simulink model "mavsim_chap5"  (R2016a)
settings: Solver=ode45  StartTime=0.0  StopTime=10000  RelTol=1e-3
InitFcn:
  | param
values from neighbouring files (symbols this model uses):
  P = GenCoefs(P)    [param.m]    (also in param_chap5.m)
undefined symbols (not defined in the file or in its folder): airdata, drawAircraft, forces_moments, plotmavstatevariables, u_trim
settings Model: Creator=beard  LastModifiedBy=Brian Jackson
settings DataIOCC: LimitDataPoints=on  SaveFormat=Array  SignalLoggingSaveFormat=ModelDataLogs
settings OptimizationCC: ExpressionDepthLimit=2147483647  InitFltsAndDblsToZero=on
settings DebuggingCC: UnderspecifiedInitializationDetection=Classic  MergeDetectMultiDrivingBlocksExec=none  SolverPrmCheckMsg=warning  FcnCallInpInsideContextMsg=UseLocalSettings  StateNameClashWarn=warning
settings HardwareCC: ProdBitPerPointer=32  ProdLargestAtomicFloat=None  ProdIntDivRoundTo=Undefined  ProdEndianess=Unspecified  ProdWordSize=32  ProdHWDeviceType=32-bit Generic
settings ModelReferenceCC: PropagateSignalLabelsOutOfModel=off
settings GRTTargetCC: CombineOutputUpdateFcns=off  GRTInterface=on
settings ConfigComp: CovModelRefEnable=Off  CovSFcnEnable=off

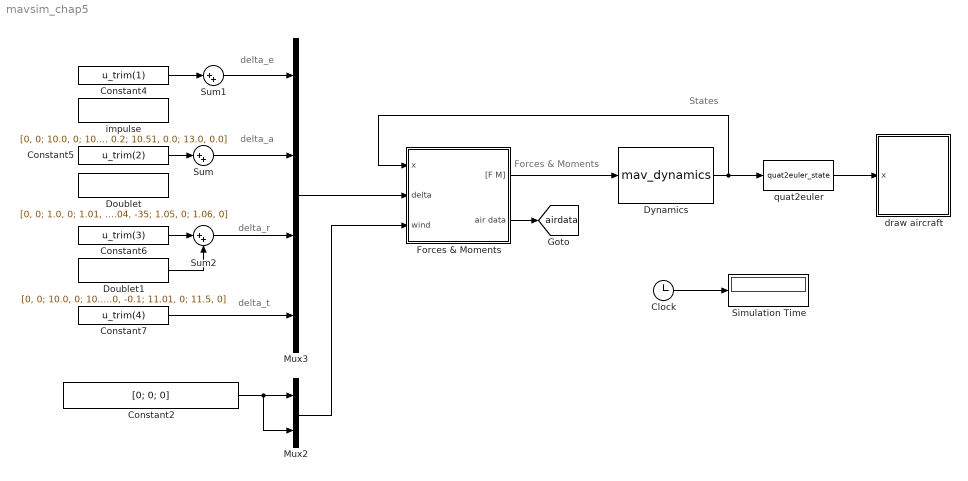
== system mavsim_chap5 ==
  note: delta_r
  note: delta_t
  note: Forces & Moments
  note: States
  note: delta_e
  note: delta_a
  Clock : Clock
  Constant2 : Constant  Value=[0; 0; 0]
  Constant4 : Constant  Value=u_trim(1)
  Constant5 : Constant  Value=u_trim(2)
  Constant6 : Constant  Value=u_trim(3)
  Constant7 : Constant  Value=u_trim(4)
  Doublet : FromWorkspace  VariableName=[0, 0; 1.0, 0; 1.01, 35; 1.02, 35; 1.03, -35; 1.04, -35; 1.05, 0; 1.06, 0]  SampleTime=0
  Doublet1 : FromWorkspace  VariableName=[0, 0; 10.0, 0; 10.01, 0.1; 10.5, 0.1; 10.51, -0.1; 11.0, -0.1; 11.01, 0; 11.5, 0]  SampleTime=0
  Dynamics : S-Function  FunctionName=mav_dynamics  Parameters=P  SFunctionDeploymentMode=off  EnableBusSupport=off
  Forces & Moments : Subsystem
  Mux2 : Mux  Inputs=2
  Mux3 : Mux
  Simulation Time : Display
  Sum : Sum  Inputs=|++
  Sum1 : Sum  Inputs=|++
  Sum2 : Sum  Inputs=|++
  draw aircraft : Subsystem
      mask Display: image(imread('tv.jpg'))
  impulse : FromWorkspace  VariableName=[0, 0; 10.0, 0; 10.01, 0.2; 10.5, 0.2; 10.51, 0.0; 13.0, 0.0]  SampleTime=0
  "quat2euler " : MATLABFcn  MATLABFcn=quat2euler_state
  tag scope: airdata=global
  wires:
  Dynamics/1 -> "quat2euler "/1, Forces & Moments/1(x)
  Forces & Moments/1("[F M]") -> Dynamics/1
  Clock/1 -> Simulation Time/1
  Forces & Moments/2(air data) -> [airdata]
  Constant2/1 -> Mux2/1, Mux2/2
  Constant5/1 -> Sum/1
  Constant4/1 -> Sum1/1
  Constant6/1 -> Sum2/1
  Mux3/1 -> Forces & Moments/2(delta)
  Mux2/1 -> Forces & Moments/3(wind)
  Sum1/1 -> Mux3/1
  Sum/1 -> Mux3/2
  Sum2/1 -> Mux3/3
  Constant7/1 -> Mux3/4
  "quat2euler "/1 -> draw aircraft/1(x)
  Doublet1/1 -> Sum2/2

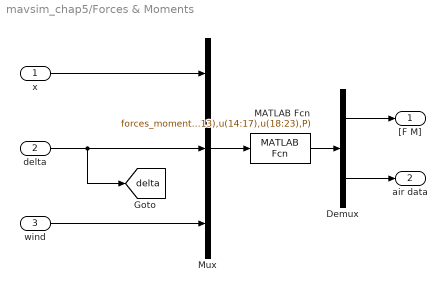
== system mavsim_chap5/Forces & Moments ==
  x : Inport
  delta : Inport  Port=2
  wind : Inport  Port=3
  Demux : Demux  Outputs=[6;6]
  MATLAB Fcn : MATLABFcn  MATLABFcn=forces_moments(u(1:13),u(14:17),u(18:23),P)  OutputDimensions=12
  Mux : Mux  Inputs=3
  "[F M]" : Outport
  air data : Outport  Port=2
  tag scope: delta=global
  wires:
  x/1 -> Mux/1
  delta/1 -> [delta], Mux/2
  wind/1 -> Mux/3
  MATLAB Fcn/1 -> Demux/1
  Demux/1 -> "[F M]"/1
  Mux/1 -> MATLAB Fcn/1
  Demux/2 -> air data/1

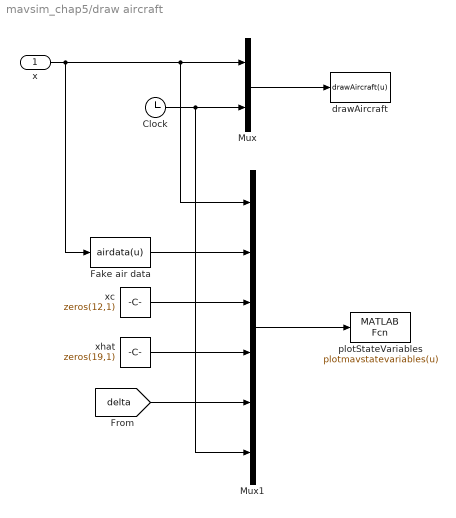
== system mavsim_chap5/draw aircraft ==
  x : Inport
  Clock : Clock
  Fake air data : MATLABFcn  MATLABFcn=airdata(u)  OutputDimensions=6  SampleTime=0.1
  Mux : Mux  Inputs=2
  Mux1 : Mux  Inputs=6
  drawAircraft : MATLABFcn  MATLABFcn=drawAircraft(u)  OutputDimensions=0  SampleTime=0.1
  plotStateVariables : MATLABFcn  MATLABFcn=plotmavstatevariables(u)  OutputDimensions=0  SampleTime=0.1
  xc : Constant  Value=zeros(12,1)
  xhat : Constant  Value=zeros(19,1)
  wires:
  Fake air data/1 -> Mux1/2
  [delta] -> Mux1/5
  xc/1 -> Mux1/3
  xhat/1 -> Mux1/4
  Mux1/1 -> plotStateVariables/1
  Clock/1 -> Mux1/6, Mux/2
  x/1 -> Fake air data/1, Mux1/1, Mux/1
  Mux/1 -> drawAircraft/1
